simulink model "COM37268D1Example"  (R2021b)
settings: Solver=FixedStepAuto  StartTime=0.0  StopTime=inf  FixedStep=0.001  RelTol=1e-3
undefined symbols (not defined in the file): canChannel
libraries: canlib x2, canmsglib x1, sldrtlib x1
settings Model: Creator=linsh  LastModifiedBy=ROMA_PC_4
settings RTWCC: Description=Simulink Desktop Real-Time  SystemTargetFile=sldrt.tlc  TemplateMakefile=sldrt.tmf  TargetLang=C++  RTWCompilerOptimization=on
settings CodeAppCC: MaxIdLength=95
settings SimulinkDesktopRealTimeCC: TargetPreCompLibLocation=C:\Tools\Mathworks\toolbox\sldrt\lib\win64  TargetLangStandard=C++11 (ISO)

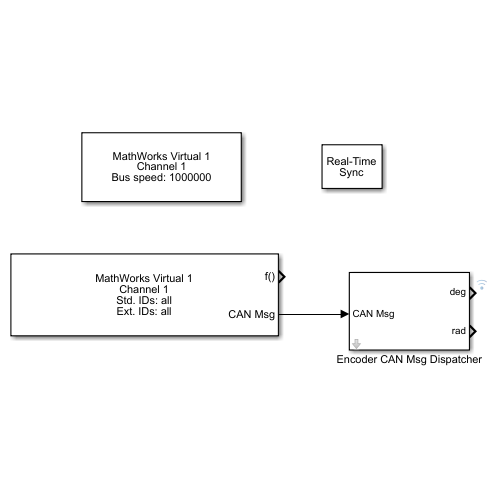
[thumbnail: Simulink's stored preview of the top-level diagram]
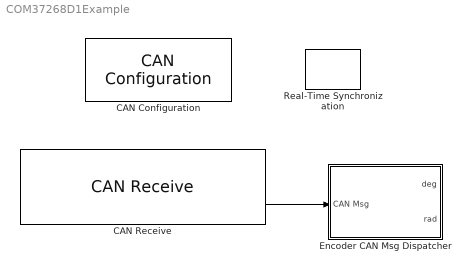
== system COM37268D1Example ==
  CAN Configuration : canlib/CAN Configuration  BlockHandle=37.0001  Device=MathWorks Virtual 1 (Channel 1)  DeviceMenu=MathWorks Virtual 1 (Channel 1)  ObjConstructor=canChannel('MathWorks', 'Virtual 1', 1)  BusSpeed=1000000  EnableBitParameters=off  AckMode=Normal
      settings: SourceProductBaseCode=VN
  CAN Receive : canlib/CAN Receive  BlockHandle=38.0001  Device=MathWorks Virtual 1 (Channel 1)  DeviceMenu=MathWorks Virtual 1 (Channel 1)  ObjConstructor=canChannel('MathWorks', 'Virtual 1', 1)  EnableStandardIDsFilter=off  StdIDsCombo=Allow all  StandardIDs=0  EnableExtendedIDsFilter=off  ExtIDsCombo=Allow all  ExtendedIDs=0  SampleTime=0.001  MsgsPerTimestep=all  InternalFilterUpdateStatus=on  BusOutput=off
      settings: SourceProductBaseCode=VN
  Encoder CAN Msg Dispatcher : Subsystem  mask{ID=1}
      mask prompts: ID "CAN std ID"
  Real-Time Synchronization : sldrtlib/Real-Time Synchronization  SampleTime=0.001  MaxMissedTicks=1000  ShowMissedTicks=off  YieldWhenWaiting=off
  wires:
  CAN Receive/2 -> Encoder CAN Msg Dispatcher/1(CAN Msg)

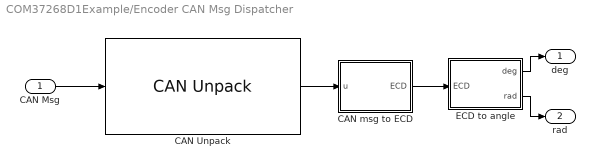
== system COM37268D1Example/Encoder CAN Msg Dispatcher ==
  CAN Msg : Inport
  CAN Unpack : canmsglib/CAN Unpack  MsgList=(none)  MsgName=CAN Msg  MsgIDType=Standard (11-bit identifier)  MsgIdentifier=ID  MsgLength=7  SignalInfo={}  IDPort=off  TimestampPort=off  ErrorPort=off  RemotePort=off  LengthPort=off  StatusPort=off  ApplyMinMax=off
      settings: SourceProductBaseCode=ME,XP,VN  DataFormat=raw data
  CAN msg to ECD : MATLAB Function  TreatAsAtomicUnit=on
  ECD to angle : MATLAB Function  TreatAsAtomicUnit=on
  deg : Outport
  rad : Outport  Port=2
  wires:
  CAN Unpack/1 -> CAN msg to ECD/1(u)
  CAN msg to ECD/1(ECD) -> ECD to angle/1(ECD)
  ECD to angle/1(deg) -> deg/1
  ECD to angle/2(rad) -> rad/1
  CAN Msg/1 -> CAN Unpack/1

== matlab function COM37268D1Example/Encoder CAN Msg Dispatcher/ECD to angle ==
  data: ECD input; deg output; rad output
function [deg,rad]= fcn(ECD)
deg = double(ECD) / 32768.0 * 360.0;
rad = double(ECD) / 32768.0 * 2.0 * pi;

== matlab function COM37268D1Example/Encoder CAN Msg Dispatcher/CAN msg to ECD ==
  data: u input; ECD output
function ECD  = fcn(u)
u=uint8(u);
length = u(1);
ID = u(2);
cmd = u(3);
ECD = uint16(0);
ECD=typecast([u(4) u(5)],'uint16');
